simulink model "Example3_Calibrating_The_AR_Drone"  (R2016a)
settings: configuration reference "AR_Drone_ConfigSet" (kept outside this file)
undefined symbols (not defined in the file or in its folder): Accel_Calib_Gain, Accel_Calib_Offset, DiscIntNeverNeededParam, Mag_Calib_Gain_Vector, Mag_Calib_Offset_Vector
libraries: simulink x5, vrlib x2, AR_Drone_2_Library x1
(part 1 of 2)
settings Model: SimulationMode=external  Creator=sannem  LastModifiedBy=sannem
settings ConfigSetRef: SourceLocation=Base Workspace

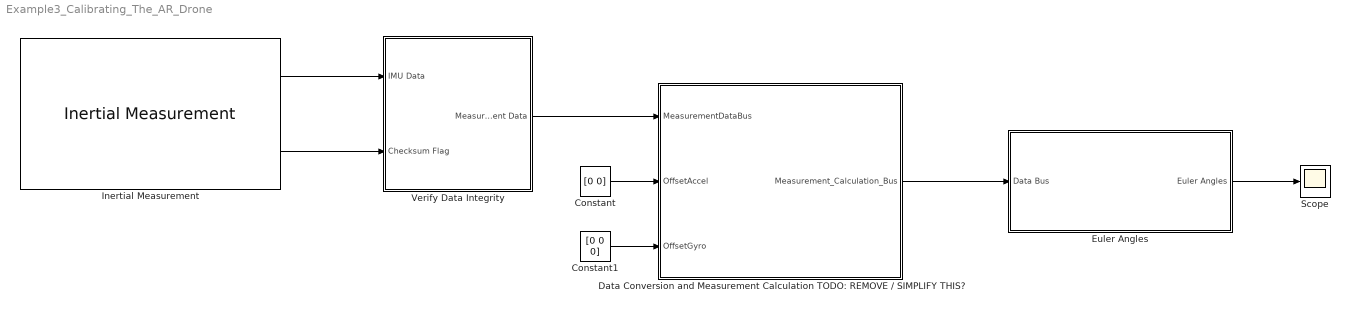
== system Example3_Calibrating_The_AR_Drone ==
  Constant : Constant  Value=[0 0]
  Constant1 : Constant  Value=[0 0 0]
  Data Conversion and Measurement Calculation TODO: REMOVE / SIMPLIFY THIS? : Subsystem
  Euler Angles : Subsystem
  Inertial Measurement : AR_Drone_2_Library/Inertial Measurement  Ts=1/400
  Scope : Scope
  Verify Data Integrity : Subsystem
  wires:
  Euler Angles/1(Euler Angles) -> Scope/1
  Constant/1 -> Data Conversion and Measurement Calculation TODO: REMOVE / SIMPLIFY THIS?/2(OffsetAccel)
  Data Conversion and Measurement Calculation TODO: REMOVE / SIMPLIFY THIS?/1(Measurement_Calculation_Bus) -> Euler Angles/1(Data Bus)
  Constant1/1 -> Data Conversion and Measurement Calculation TODO: REMOVE / SIMPLIFY THIS?/3(OffsetGyro)
  Inertial Measurement/1 -> Verify Data Integrity/1(IMU Data)
  Inertial Measurement/2 -> Verify Data Integrity/2(Checksum Flag)
  Verify Data Integrity/1(Measurement Data) -> Data Conversion and Measurement Calculation TODO: REMOVE / SIMPLIFY THIS?/1(MeasurementDataBus)

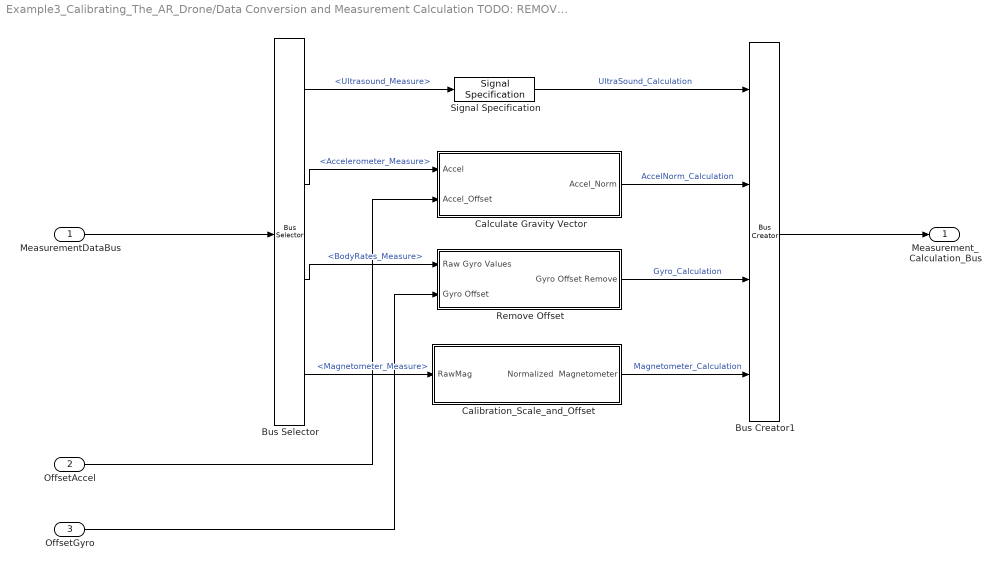
== system Example3_Calibrating_The_AR_Drone/Data Conversion and Measurement Calculation TODO: REMOVE // SIMPLIFY THIS? ==
  MeasurementDataBus : Inport
  OffsetAccel : Inport  Port=2
  OffsetGyro : Inport  Port=3
  Bus Creator1 : BusCreator  Inputs=4
  Bus Selector : BusSelector  OutputSignals=Ultrasound_Measure,Accelerometer_Measure,BodyRates_Measure,Magnetometer_Measure
  Calculate Gravity Vector : Subsystem
  Calibration_Scale_and_Offset : Subsystem
  Remove Offset : Subsystem
  Signal Specification : SignalSpecification
  Measurement_Calculation_Bus : Outport
  wires:
  MeasurementDataBus/1 -> Bus Selector/1
  Bus Selector/4 -> Calibration_Scale_and_Offset/1(RawMag)  "<Magnetometer_Measure>"
  OffsetAccel/1 -> Calculate Gravity Vector/2(Accel_Offset)
  OffsetGyro/1 -> Remove Offset/2(Gyro Offset)
  Bus Selector/3 -> Remove Offset/1(Raw Gyro Values)  "<BodyRates_Measure>"
  Bus Selector/1 -> Signal Specification/1  "<Ultrasound_Measure>"
  Calibration_Scale_and_Offset/1(Normalized  Magnetometer) -> Bus Creator1/4  "Magnetometer_Calculation"
  Remove Offset/1(Gyro Offset Remove) -> Bus Creator1/3  "Gyro_Calculation"
  Signal Specification/1 -> Bus Creator1/1  "UltraSound_Calculation"
  Calculate Gravity Vector/1(Accel_Norm) -> Bus Creator1/2  "AccelNorm_Calculation"
  Bus Creator1/1 -> Measurement_Calculation_Bus/1
  Bus Selector/2 -> Calculate Gravity Vector/1(Accel)  "<Accelerometer_Measure>"

== system Example3_Calibrating_The_AR_Drone/Euler Angles ==
  Data Bus : Inport  OutDataTypeStr=Bus: Measurement_Calculation_Bus
  Bus Selector2 : BusSelector  OutputSignals=AccelNorm_Calculation
  Bus Selector3 : BusSelector  OutputSignals=Gyro_Calculation
  Compute Euler Angles : Subsystem
  Invert : Gain  Gain=-1
  Mux : Mux  Inputs=3
  Euler Angles : Outport
  wires:
  Data Bus/1 -> Bus Selector3/1, Bus Selector2/1
  Bus Selector3/1 -> Compute Euler Angles/2(Gyroscope Data)  "<Gyro_Calculation>"
  Bus Selector2/1 -> Compute Euler Angles/1(Accelerometer Data)  "<AccelNorm_Calculation>"
  Compute Euler Angles/1(Filtered Roll) -> Mux/1
  Compute Euler Angles/2(Filtered Pitch) -> Mux/2
  Compute Euler Angles/3(Yaw) -> Mux/3
  Mux/1 -> Invert/1
  Invert/1 -> Euler Angles/1

== system Example3_Calibrating_The_AR_Drone/Verify Data Integrity ==
  IMU Data : Inport
  Checksum Flag : Inport  Port=2
  Bus Creator1 : BusCreator  Inputs=5
  CheckSum Pre-Processing : Subsystem  TreatAsAtomicUnit=on
      settings: RTWSystemCode=Inline
  Measurement Data : Outport
  wires:
  CheckSum Pre-Processing/2(Magnetometer_Measure) -> Bus Creator1/2  "Magnetometer_Measure"
  Bus Creator1/1 -> Measurement Data/1  "RawMeasurement_DataBus"
  CheckSum Pre-Processing/3(BodyRates_Measure) -> Bus Creator1/3  "BodyRates_Measure"
  CheckSum Pre-Processing/1(UltraSoundHeight_Measure) -> Bus Creator1/1  "Ultrasound_Measure"
  Checksum Flag/1 -> CheckSum Pre-Processing/2(CheckSumFlag)
  IMU Data/1 -> CheckSum Pre-Processing/1(IMU Packets)
  CheckSum Pre-Processing/5(GyroTemp_Measure) -> Bus Creator1/5  "GyroTemp_Measure"
  CheckSum Pre-Processing/4(Accelerometer_Measure) -> Bus Creator1/4  "Accelerometer_Measure"

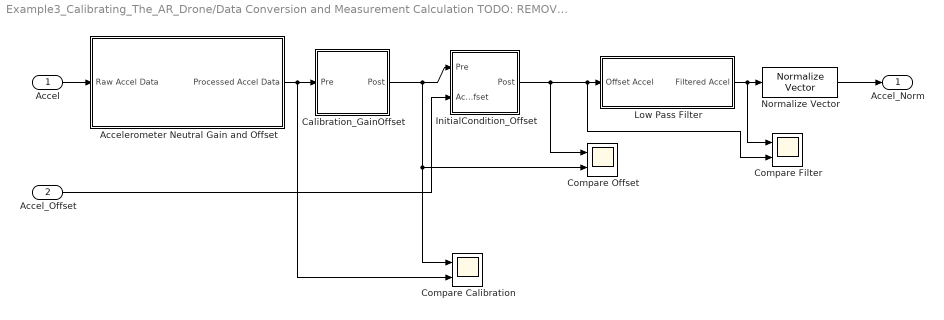
== system Example3_Calibrating_The_AR_Drone/Data Conversion and Measurement Calculation TODO: REMOVE // SIMPLIFY THIS?/Calculate Gravity Vector ==
  Accel : Inport
  Accel_Offset : Inport  Port=2
  Accelerometer Neutral Gain and Offset : Subsystem
  Calibration_GainOffset : Subsystem
  Compare Calibration : Scope  NumInputPorts=2
  Compare Filter : Scope  NumInputPorts=2
  Compare Offset : Scope  NumInputPorts=2
  InitialCondition_Offset : Subsystem
  Low Pass Filter : Subsystem
  Normalize Vector : vrlib/Utilities/Normalize Vector  maxzero=0
  Accel_Norm : Outport
  wires:
  Accel_Offset/1 -> InitialCondition_Offset/2(Accel_Offset)
  Accelerometer Neutral Gain and Offset/1(Processed Accel Data) -> Compare Calibration/2, Calibration_GainOffset/1(Pre)
  Calibration_GainOffset/1(Post) -> Compare Offset/2, Compare Calibration/1, InitialCondition_Offset/1(Pre)
  Low Pass Filter/1(Filtered Accel) -> Normalize Vector/1, Compare Filter/1
  InitialCondition_Offset/1(Post) -> Low Pass Filter/1(Offset Accel), Compare Filter/2, Compare Offset/1
  Accel/1 -> Accelerometer Neutral Gain and Offset/1(Raw Accel Data)
  Normalize Vector/1 -> Accel_Norm/1

== system Example3_Calibrating_The_AR_Drone/Data Conversion and Measurement Calculation TODO: REMOVE // SIMPLIFY THIS?/Calibration_Scale_and_Offset ==
  RawMag : Inport
  Normalize Vector : vrlib/Utilities/Normalize Vector  maxzero=0
  Process Raw Mag Data : Subsystem  Variant=on  OverrideUsingVariant=TempVariantA
  Normalized  Magnetometer : Outport
  wires:
  Process Raw Mag Data/1(MagVector) -> Normalize Vector/1
  RawMag/1 -> Process Raw Mag Data/1(Magnetometer)
  Normalize Vector/1 -> Normalized  Magnetometer/1

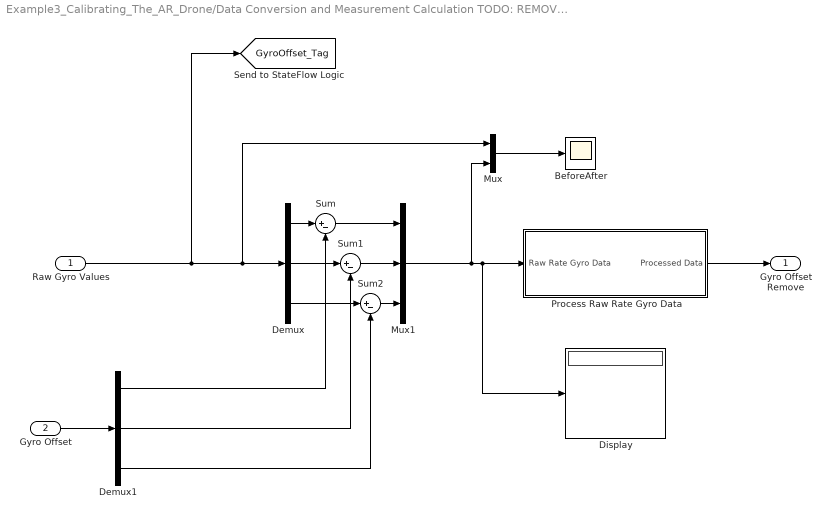
== system Example3_Calibrating_The_AR_Drone/Data Conversion and Measurement Calculation TODO: REMOVE // SIMPLIFY THIS?/Remove Offset ==
  Raw Gyro Values : Inport
  Gyro Offset : Inport  Port=2
  BeforeAfter : Scope
  Demux : Demux  Outputs=3
  Demux1 : Demux  Outputs=3
  Display : Display
  Mux : Mux  Inputs=2
  Mux1 : Mux  Inputs=3
  Process Raw Rate Gyro Data : Subsystem
  Sum : Sum  Inputs=|+-
  Sum1 : Sum  Inputs=|+-
  Sum2 : Sum  Inputs=|+-
  Gyro Offset Remove : Outport
  tag scope: GyroOffset_Tag=global
  wires:
  Process Raw Rate Gyro Data/1(Processed Data) -> Gyro Offset Remove/1
  Mux/1 -> BeforeAfter/1
  Raw Gyro Values/1 -> Demux/1, Mux/1, [GyroOffset_Tag]
  Gyro Offset/1 -> Demux1/1
  Mux1/1 -> Process Raw Rate Gyro Data/1(Raw Rate Gyro Data), Display/1, Mux/2
  Demux1/3 -> Sum2/2
  Demux1/2 -> Sum1/2
  Demux1/1 -> Sum/2
  Demux/2 -> Sum1/1
  Demux/1 -> Sum/1
  Sum1/1 -> Mux1/2
  Demux/3 -> Sum2/1
  Sum2/1 -> Mux1/3
  Sum/1 -> Mux1/1

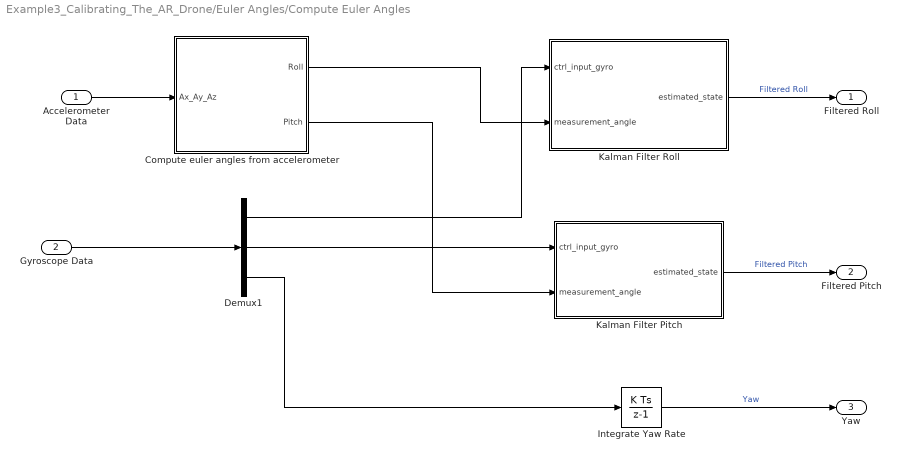
== system Example3_Calibrating_The_AR_Drone/Euler Angles/Compute Euler Angles ==
  Accelerometer Data : Inport
  Gyroscope Data : Inport  Port=2
  Compute euler angles from accelerometer : MATLAB Function  TreatAsAtomicUnit=on
  Demux1 : Demux  Outputs=3
  Integrate Yaw Rate : DiscreteIntegrator  SampleTime=1/400  OutDataTypeStr=double  ICPrevOutput=DiscIntNeverNeededParam  ICPrevScaledInput=DiscIntNeverNeededParam
  Kalman Filter Pitch : MATLAB Function  TreatAsAtomicUnit=on
  Kalman Filter Roll : MATLAB Function  TreatAsAtomicUnit=on
  Filtered Roll : Outport
  Filtered Pitch : Outport  Port=2
  Yaw : Outport  Port=3
  wires:
  Compute euler angles from accelerometer/2(Pitch) -> Kalman Filter Pitch/2(measurement_angle)
  Integrate Yaw Rate/1 -> Yaw/1  "Yaw"
  Kalman Filter Roll/1(estimated_state) -> Filtered Roll/1  "Filtered Roll"
  Demux1/3 -> Integrate Yaw Rate/1
  Demux1/2 -> Kalman Filter Pitch/1(ctrl_input_gyro)
  Kalman Filter Pitch/1(estimated_state) -> Filtered Pitch/1  "Filtered Pitch"
  Demux1/1 -> Kalman Filter Roll/1(ctrl_input_gyro)
  Compute euler angles from accelerometer/1(Roll) -> Kalman Filter Roll/2(measurement_angle)
  Accelerometer Data/1 -> Compute euler angles from accelerometer/1(Ax_Ay_Az)
  Gyroscope Data/1 -> Demux1/1

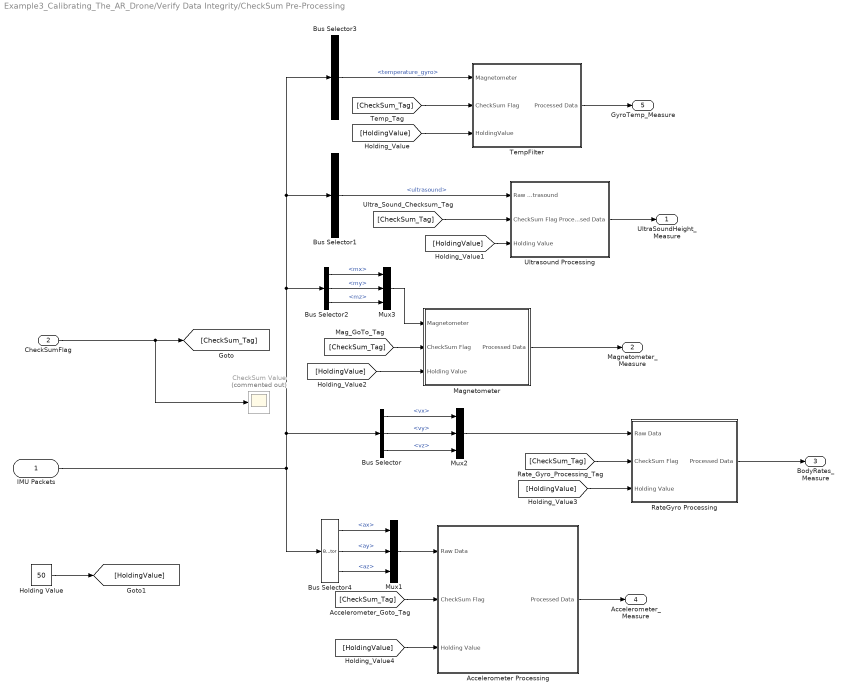
== system Example3_Calibrating_The_AR_Drone/Verify Data Integrity/CheckSum Pre-Processing ==
  IMU Packets : Inport
  CheckSumFlag : Inport  Port=2
  Accelerometer Processing : Subsystem
  Bus Selector : BusSelector  OutputSignals=vx,vy,vz
  Bus Selector1 : BusSelector  OutputSignals=ultrasound
  Bus Selector2 : BusSelector  OutputSignals=mx,my,mz
  Bus Selector3 : BusSelector  OutputSignals=temperature_gyro
  Bus Selector4 : BusSelector  OutputSignals=ax,ay,az
  CheckSum Value : Scope  Commented=on
  Holding Value : Constant  Value=50
  Magnetometer : Subsystem
  Mux1 : Mux  Inputs=3
  Mux2 : Mux  Inputs=3
  Mux3 : Mux  Inputs=3
  RateGyro Processing : Subsystem
  TempFilter : Subsystem
  Ultrasound Processing : Subsystem
  UltraSoundHeight_Measure : Outport
  Magnetometer_Measure : Outport  Port=2
  BodyRates_Measure : Outport  Port=3
  Accelerometer_Measure : Outport  Port=4
  GyroTemp_Measure : Outport  Port=5
  wires:
  Mux3/1 -> Magnetometer/1(Magnetometer)
  Holding Value/1 -> [HoldingValue]
  [HoldingValue] -> Accelerometer Processing/3(Holding Value)
  [HoldingValue] -> RateGyro Processing/3(Holding Value)
  [HoldingValue] -> Magnetometer/3(Holding Value)
  [HoldingValue] -> Ultrasound Processing/3(Holding Value)
  [HoldingValue] -> TempFilter/3(HoldingValue)
  [CheckSum_Tag] -> TempFilter/2(CheckSum Flag)
  TempFilter/1(Processed Data) -> GyroTemp_Measure/1
  Bus Selector3/1 -> TempFilter/1(Magnetometer)  "<temperature_gyro>"
  Bus Selector/3 -> Mux2/3  "<vz>"
  Bus Selector/2 -> Mux2/2  "<vy>"
  Bus Selector/1 -> Mux2/1  "<vx>"
  Ultrasound Processing/1(Processed Data) -> UltraSoundHeight_Measure/1
  [CheckSum_Tag] -> Accelerometer Processing/2(CheckSum Flag)
  Magnetometer/1(Processed Data) -> Magnetometer_Measure/1
  [CheckSum_Tag] -> Magnetometer/2(CheckSum Flag)
  Bus Selector2/3 -> Mux3/3  "<mz>"
  Bus Selector2/2 -> Mux3/2  "<my>"
  Bus Selector2/1 -> Mux3/1  "<mx>"
  RateGyro Processing/1(Processed Data) -> BodyRates_Measure/1
  [CheckSum_Tag] -> RateGyro Processing/2(CheckSum Flag)
  Mux2/1 -> RateGyro Processing/1(Raw Data)
  Accelerometer Processing/1(Processed Data) -> Accelerometer_Measure/1
  [CheckSum_Tag] -> Ultrasound Processing/2(CheckSum Flag)
  Mux1/1 -> Accelerometer Processing/1(Raw Data)
  Bus Selector4/3 -> Mux1/3  "<az>"
  Bus Selector4/2 -> Mux1/2  "<ay>"
  Bus Selector4/1 -> Mux1/1  "<ax>"
  IMU Packets/1 -> Bus Selector4/1, Bus Selector2/1, Bus Selector1/1, Bus Selector3/1, Bus Selector/1
  CheckSumFlag/1 -> CheckSum Value/1, [CheckSum_Tag]
  Bus Selector1/1 -> Ultrasound Processing/1(Raw Ultrasound)  "<ultrasound>"

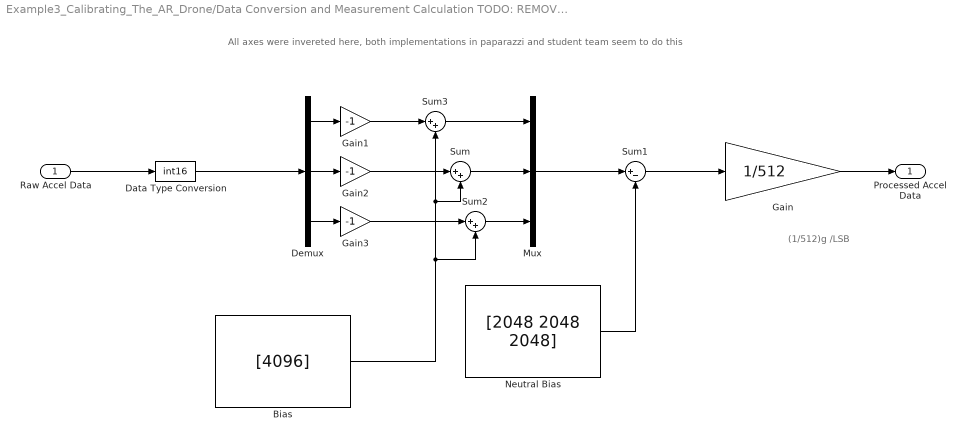
== system Example3_Calibrating_The_AR_Drone/Data Conversion and Measurement Calculation TODO: REMOVE // SIMPLIFY THIS?/Calculate Gravity Vector/Accelerometer Neutral Gain and Offset ==
  note: (1/512)g /LSB
  note: All axes were invereted here, both implementations in paparazzi and student team seem to do this
  Raw Accel Data : Inport
  Bias : Constant  Value=[4096]
  Data Type Conversion : DataTypeConversion  OutDataTypeStr=int16
  Demux : Demux  Outputs=3
  Gain : Gain  Gain=1/512
  Gain1 : Gain  Gain=-1  OutDataTypeStr=double
  Gain2 : Gain  Gain=-1  OutDataTypeStr=double
  Gain3 : Gain  Gain=-1  OutDataTypeStr=double
  Mux : Mux  Inputs=3
  Neutral Bias : Constant  Value=[2048 2048 2048]
  Sum : Sum  Inputs=|++
  Sum1 : Sum  Inputs=|+-
  Sum2 : Sum  Inputs=|++
  Sum3 : Sum  Inputs=|++
  Processed Accel Data : Outport
  wires:
  Gain1/1 -> Sum3/1
  Data Type Conversion/1 -> Demux/1
  Bias/1 -> Sum3/2, Sum/2, Sum2/2
  Sum2/1 -> Mux/3
  Gain3/1 -> Sum2/1
  Demux/3 -> Gain3/1
  Sum/1 -> Mux/2
  Gain2/1 -> Sum/1
  Demux/2 -> Gain2/1
  Sum3/1 -> Mux/1
  Demux/1 -> Gain1/1
  Raw Accel Data/1 -> Data Type Conversion/1
  Neutral Bias/1 -> Sum1/2
  Mux/1 -> Sum1/1
  Gain/1 -> Processed Accel Data/1
  Sum1/1 -> Gain/1

== system Example3_Calibrating_The_AR_Drone/Data Conversion and Measurement Calculation TODO: REMOVE // SIMPLIFY THIS?/Calculate Gravity Vector/Calibration_GainOffset ==
  Pre : Inport
  Accel_Calib_Gain : Constant  Value=[Accel_Calib_Gain.Gain_X Accel_Calib_Gain.Gain_Y Accel_Calib_Gain.Gain_Z]
      settings: AttributesFormatString=%<Value>
  Accel_Calib_Offset : Constant  Value="[Accel_Calib_Offset.Gain_X  Accel_Calib_Offset.Gain_Y  Accel_Calib_Offset.Gain_Z]"
      settings: AttributesFormatString=%<Value>
  Gain : Gain  Gain=-1  OutDataTypeStr=Inherit: Same as input
  Multiply : Product  Inputs=*/
  Sum : Sum  Inputs=|+-
  Post : Outport
  wires:
  Gain/1 -> Multiply/2
  Accel_Calib_Gain/1 -> Gain/1
  Pre/1 -> Sum/1
  Sum/1 -> Multiply/1
  Accel_Calib_Offset/1 -> Sum/2
  Multiply/1 -> Post/1

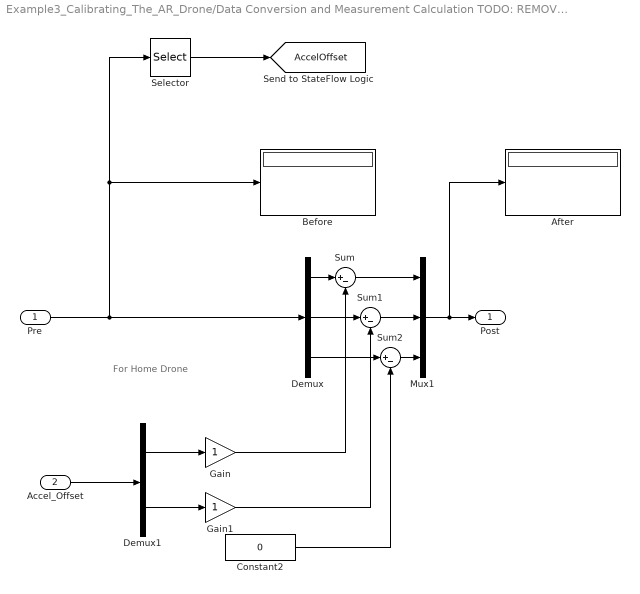
== system Example3_Calibrating_The_AR_Drone/Data Conversion and Measurement Calculation TODO: REMOVE // SIMPLIFY THIS?/Calculate Gravity Vector/InitialCondition_Offset ==
  note: For Home Drone
  Pre : Inport
  Accel_Offset : Inport  Port=2
  After : Display
  Before : Display
  Constant2 : Constant  Value=0
  Demux : Demux  Outputs=3
  Demux1 : Demux  Outputs=2
  Gain : Gain
  Gain1 : Gain
  Mux1 : Mux  Inputs=3
  Selector : Selector  InputPortWidth=3  IndexOptions=Index vector (dialog)  Indices=[1 2]  OutputSizes=1
  Sum : Sum  Inputs=|+-
  Sum1 : Sum  Inputs=|+-
  Sum2 : Sum  Inputs=|+-
  Post : Outport
  tag scope: AccelOffset=global
  wires:
  Constant2/1 -> Sum2/2
  Gain1/1 -> Sum1/2
  Gain/1 -> Sum/2
  Selector/1 -> [AccelOffset]
  Pre/1 -> Before/1, Selector/1, Demux/1
  Demux1/2 -> Gain1/1
  Demux1/1 -> Gain/1
  Accel_Offset/1 -> Demux1/1
  Mux1/1 -> After/1, Post/1
  Demux/2 -> Sum1/1
  Demux/1 -> Sum/1
  Sum1/1 -> Mux1/2
  Demux/3 -> Sum2/1
  Sum2/1 -> Mux1/3
  Sum/1 -> Mux1/1

== system Example3_Calibrating_The_AR_Drone/Data Conversion and Measurement Calculation TODO: REMOVE // SIMPLIFY THIS?/Calculate Gravity Vector/Low Pass Filter ==
  Offset Accel : Inport
  Add : Sum
  Gain : Gain  Gain=0.8
  Gain1 : Gain  Gain=0.2
  Unit Delay : UnitDelay  SampleTime=-1
  Filtered Accel : Outport
  wires:
  Offset Accel/1 -> Gain1/1
  Add/1 -> Filtered Accel/1, Unit Delay/1
  Gain/1 -> Add/2
  Gain1/1 -> Add/1
  Unit Delay/1 -> Gain/1

== system Example3_Calibrating_The_AR_Drone/Data Conversion and Measurement Calculation TODO: REMOVE // SIMPLIFY THIS?/Calibration_Scale_and_Offset/Process Raw Mag Data ==
  Magnetometer : Inport
  Process Raw Mag Data (Home_330453) : Subsystem  VariantControl=TempVariantA
  Process Raw Mag Data (Work_255725) : Subsystem  VariantControl=TempVariantB
  MagVector : Outport

== system Example3_Calibrating_The_AR_Drone/Data Conversion and Measurement Calculation TODO: REMOVE // SIMPLIFY THIS?/Remove Offset/Process Raw Rate Gyro Data ==
  note: const float Sensitivity[ 3 ] = { 0.0609 , 0.0609 , 0.0609 } ;
      | const float Neutral[ 3 ] = { 0.0 , 0.0 , 0.0 } ;
      | const int16_t Offset[ 3 ] = { - 73 , 14 , - 13 } ;
      | const int16_t Noises[ 3 ] = { 35 , 35 , 15 } ;
      |
      | int16_t vRaws[ 3 ] = {
      | Navdata :: IMU :: Gyroscope :: getRawX (),
      | Navdata :: IMU :: Gyroscope :: getRawY (),
      | Navdata :: IMU :: Gyroscope :: getRawZ ()
      | } ;
      |
      | gyroscope[i] = vRaws[i] * Gyroscope :: Sensitivity[i] * M_PI / 180.0 ;
  Raw Rate Gyro Data : Inport
  Gain : Gain  Gain=[0.0609, 0.0609, 0.0609]  ParamDataTypeStr=double
  Processed Data : Outport
  wires:
  Gain/1 -> Processed Data/1
  Raw Rate Gyro Data/1 -> Gain/1

== system Example3_Calibrating_The_AR_Drone/Verify Data Integrity/CheckSum Pre-Processing/Accelerometer Processing ==
  Raw Data : Inport
  CheckSum Flag : Inport  Port=2
  Holding Value : Inport  Port=3
  Calculate Accel Data : Subsystem  Commented=through
  CheckSum Correction : Subsystem
  Processed Data : Outport
  wires:
  Holding Value/1 -> CheckSum Correction/3(Holding Value)
  Calculate Accel Data/1(Processed Accel Data) -> CheckSum Correction/1(CalculatedData)
  CheckSum Correction/1(Pre-Processed Height) -> Processed Data/1
  Raw Data/1 -> Calculate Accel Data/1(Raw Accel Data)
  CheckSum Flag/1 -> CheckSum Correction/2(CheckSumFlag)

== system Example3_Calibrating_The_AR_Drone/Verify Data Integrity/CheckSum Pre-Processing/Magnetometer ==
  Magnetometer : Inport
  CheckSum Flag : Inport  Port=2
  Holding Value : Inport  Port=3
  CheckSum Correction : Subsystem
  Process Raw Mag Data : Subsystem  Commented=through
  Processed Data : Outport
  wires:
  Holding Value/1 -> CheckSum Correction/3(Holding Value)
  Process Raw Mag Data/1(ProcessedData) -> CheckSum Correction/1(CalculatedData)
  Magnetometer/1 -> Process Raw Mag Data/1(Magnetometer)
  CheckSum Correction/1(Pre-Processed Data) -> Processed Data/1
  CheckSum Flag/1 -> CheckSum Correction/2(CheckSumFlag)

== system Example3_Calibrating_The_AR_Drone/Verify Data Integrity/CheckSum Pre-Processing/RateGyro Processing ==
  Raw Data : Inport
  CheckSum Flag : Inport  Port=2
  Holding Value : Inport  Port=3
  CheckSum Correction : Subsystem
  Process Data : Subsystem  Commented=through
  Processed Data : Outport
  wires:
  Holding Value/1 -> CheckSum Correction/3(Holding Value)
  Process Data/1(Processed Data) -> CheckSum Correction/1(CalculatedData)
  Raw Data/1 -> Process Data/1(Raw Data)
  CheckSum Correction/1(Pre-Processed Height) -> Processed Data/1
  CheckSum Flag/1 -> CheckSum Correction/2(CheckSumFlag)

== system Example3_Calibrating_The_AR_Drone/Verify Data Integrity/CheckSum Pre-Processing/TempFilter ==
  Magnetometer : Inport
  CheckSum Flag : Inport  Port=2
  HoldingValue : Inport  Port=3
  CheckSum Correction : Subsystem
  Process Raw Mag Data : Subsystem  Commented=through
  Processed Data : Outport
  wires:
  HoldingValue/1 -> CheckSum Correction/3(Holding Value)
  Process Raw Mag Data/1(ProcessedData) -> CheckSum Correction/1(CalculatedData)
  Magnetometer/1 -> Process Raw Mag Data/1(Magnetometer)
  CheckSum Correction/1(Pre-Processed Data) -> Processed Data/1
  CheckSum Flag/1 -> CheckSum Correction/2(CheckSumFlag)

== system Example3_Calibrating_The_AR_Drone/Verify Data Integrity/CheckSum Pre-Processing/Ultrasound Processing ==
  note: '192.168.1.1' 1 17725
  Raw Ultrasound : Inport
  CheckSum Flag : Inport  Port=2
  Holding Value : Inport  Port=3
  CheckSum Correction : Subsystem
  Data Type Conversion1 : DataTypeConversion
  Delay1 : Delay  DelayLength=1  InitialCondition=0
  Height Calculation : MATLAB Function  TreatAsAtomicUnit=on
  Saturation1 : Saturate  UpperLimit=100e3  LowerLimit=0
  Processed Data : Outport
  wires:
  Holding Value/1 -> CheckSum Correction/3(Holding Value)
  Saturation1/1 -> Processed Data/1
  CheckSum Correction/1(Pre-Processed Height) -> Saturation1/1
  CheckSum Flag/1 -> CheckSum Correction/2(CheckSumFlag)
  Height Calculation/1(y) -> CheckSum Correction/1(CalculatedData)
  Raw Ultrasound/1 -> Data Type Conversion1/1
  Height Calculation/2(prev_good_height) -> Delay1/1
  Data Type Conversion1/1 -> Height Calculation/1(u)
  Delay1/1 -> Height Calculation/2(z_1)

== system Example3_Calibrating_The_AR_Drone/Data Conversion and Measurement Calculation TODO: REMOVE // SIMPLIFY THIS?/Calibration_Scale_and_Offset/Process Raw Mag Data/Process Raw Mag Data (Home_330453) ==
  note: magnetometer[ 0 ] = - ( float ) navdata.mx ;
      | magnetometer[ 1 ] = ( float ) navdata.my ;
      | magnetometer[ 2 ] = - ( float ) navdata.mz ;
      | const float Sensitivity[ 3 ] = { 0.0071492608 , 0.0070882491 , 0.0074057781 } ;
      | const float Neutral[ 3 ] = { 118.0 , - 65.0 , 110.0 } ;
  Magnetometer : Inport
  Bias : Constant  Commented=on  Value=[-23 4.3 1.44]
  Constant : Constant  Value=[Mag_Calib_Offset_Vector.Gain_X Mag_Calib_Offset_Vector.Gain_Y Mag_Calib_Offset_Vector.Gain_Z]
      settings: AttributesFormatString=%<Value>
  Constant1 : Constant  Value=[Mag_Calib_Gain_Vector.Gain_X Mag_Calib_Gain_Vector.Gain_Y Mag_Calib_Gain_Vector.Gain_Z]
      settings: AttributesFormatString=%<Value>
  Divide : Product  Inputs=/*
  Sum : Sum  Inputs=|+-
  postGain : Gain  Commented=on  Gain=1./[187 163 139]
  MagVector : Outport
  wires:
  Constant1/1 -> Divide/1
  Sum/1 -> Divide/2
  Magnetometer/1 -> Sum/1
  Constant/1 -> Sum/2
  Divide/1 -> MagVector/1

== system Example3_Calibrating_The_AR_Drone/Data Conversion and Measurement Calculation TODO: REMOVE // SIMPLIFY THIS?/Calibration_Scale_and_Offset/Process Raw Mag Data/Process Raw Mag Data (Work_255725) ==
  note: 158 145 136
  note: magnetometer[ 0 ] = - ( float ) navdata.mx ;
      | magnetometer[ 1 ] = ( float ) navdata.my ;
      | magnetometer[ 2 ] = - ( float ) navdata.mz ;
      | const float Sensitivity[ 3 ] = { 0.0071492608 , 0.0070882491 , 0.0074057781 } ;
      | const float Neutral[ 3 ] = { 118.0 , - 65.0 , 110.0 } ;
  Magnetometer : Inport
  Bias : Constant  Value=[2.93 18.9 77.5]
  Low Pass Filter1 : Subsystem  Commented=through
      mask Display: disp(['Elliptic Filter with 20 Hz corner', '\n', '44 dB stopband.'])
  Sum : Sum  Inputs=|+-
  postGain : Gain  Gain=1./[167 135 132]
  preGain : Gain  Commented=through  Gain=[1 1 1]
  MagVector : Outport
  wires:
  postGain/1 -> Low Pass Filter1/1(Input)
  Magnetometer/1 -> preGain/1
  Sum/1 -> postGain/1
  preGain/1 -> Sum/1
  Bias/1 -> Sum/2
  Low Pass Filter1/1(Output) -> MagVector/1

== system Example3_Calibrating_The_AR_Drone/Verify Data Integrity/CheckSum Pre-Processing/Accelerometer Processing/Calculate Accel Data ==
  Raw Accel Data : Inport
  Bias : Constant  Value=[0 4096 4096]
  Gain : Gain  Gain=[0.001953125, 0.001953125, 0.001953125]
  Neutral Bias : Constant  Value=[2048 2048 2048]
  Sum : Sum  Inputs=|-+
  Sum1 : Sum  Inputs=|+-
  Processed Accel Data : Outport
  wires:
  Bias/1 -> Sum/2
  Neutral Bias/1 -> Sum1/2
  Sum/1 -> Sum1/1
  Gain/1 -> Processed Accel Data/1
  Sum1/1 -> Gain/1
  Raw Accel Data/1 -> Sum/1

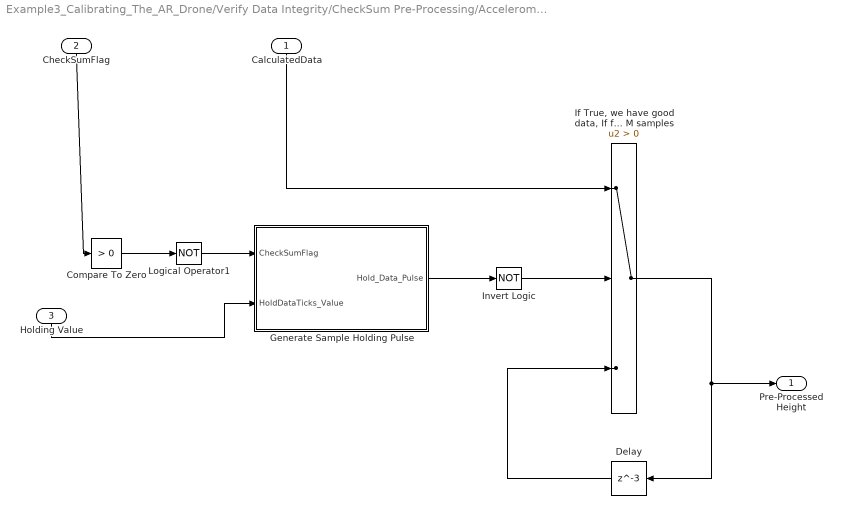
== system Example3_Calibrating_The_AR_Drone/Verify Data Integrity/CheckSum Pre-Processing/Accelerometer Processing/CheckSum Correction ==
  CalculatedData : Inport
  CheckSumFlag : Inport  Port=2
  Holding Value : Inport  Port=3
  Compare To Zero : simulink/Logic and Bit Operations/Compare To Zero  relop=>  OutDataTypeStr=boolean
  Delay : Delay  DelayLength=3  InitialCondition=0
  Generate Sample Holding Pulse : Subsystem
  "If True, we have good data, If false, we have bad data, With bad data, use previous good data from N samples ago and hold it on that value for M samples" : Switch  Criteria=u2 > Threshold
  Invert Logic : Logic  Operator=NOT  AllPortsSameDT=off  OutDataTypeStr=boolean
  Logical Operator1 : Logic  Operator=NOT  AllPortsSameDT=off  OutDataTypeStr=boolean
  Pre-Processed Height : Outport
  wires:
  Holding Value/1 -> Generate Sample Holding Pulse/2(HoldDataTicks_Value)
  Invert Logic/1 -> "If True, we have good data, If false, we have bad data, With bad data, use previous good data from N samples ago and hold it on that value for M samples"/2
  Logical Operator1/1 -> Generate Sample Holding Pulse/1(CheckSumFlag)
  Generate Sample Holding Pulse/1(Hold_Data_Pulse) -> Invert Logic/1
  Compare To Zero/1 -> Logical Operator1/1
  Delay/1 -> "If True, we have good data, If false, we have bad data, With bad data, use previous good data from N samples ago and hold it on that value for M samples"/3
  "If True, we have good data, If false, we have bad data, With bad data, use previous good data from N samples ago and hold it on that value for M samples"/1 -> Delay/1, Pre-Processed Height/1
  CalculatedData/1 -> "If True, we have good data, If false, we have bad data, With bad data, use previous good data from N samples ago and hold it on that value for M samples"/1
  CheckSumFlag/1 -> Compare To Zero/1

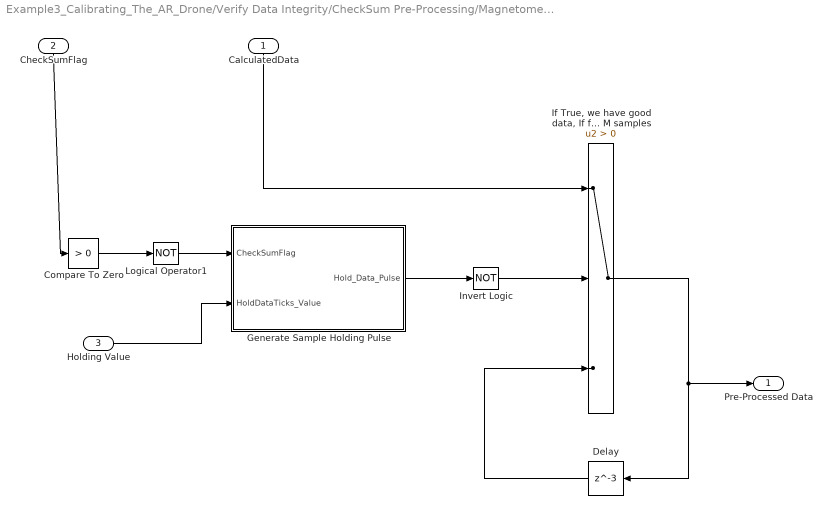
== system Example3_Calibrating_The_AR_Drone/Verify Data Integrity/CheckSum Pre-Processing/Magnetometer/CheckSum Correction ==
  CalculatedData : Inport
  CheckSumFlag : Inport  Port=2
  Holding Value : Inport  Port=3
  Compare To Zero : simulink/Logic and Bit Operations/Compare To Zero  relop=>  OutDataTypeStr=boolean
  Delay : Delay  DelayLength=3  InitialCondition=0
  Generate Sample Holding Pulse : Subsystem
  "If True, we have good data, If false, we have bad data, With bad data, use previous good data from N samples ago and hold it on that value for M samples" : Switch  Criteria=u2 > Threshold
  Invert Logic : Logic  Operator=NOT  AllPortsSameDT=off  OutDataTypeStr=boolean
  Logical Operator1 : Logic  Operator=NOT  AllPortsSameDT=off  OutDataTypeStr=boolean
  Pre-Processed Data : Outport
  wires:
  Holding Value/1 -> Generate Sample Holding Pulse/2(HoldDataTicks_Value)
  Invert Logic/1 -> "If True, we have good data, If false, we have bad data, With bad data, use previous good data from N samples ago and hold it on that value for M samples"/2
  Logical Operator1/1 -> Generate Sample Holding Pulse/1(CheckSumFlag)
  Generate Sample Holding Pulse/1(Hold_Data_Pulse) -> Invert Logic/1
  Compare To Zero/1 -> Logical Operator1/1
  Delay/1 -> "If True, we have good data, If false, we have bad data, With bad data, use previous good data from N samples ago and hold it on that value for M samples"/3
  "If True, we have good data, If false, we have bad data, With bad data, use previous good data from N samples ago and hold it on that value for M samples"/1 -> Delay/1, Pre-Processed Data/1
  CalculatedData/1 -> "If True, we have good data, If false, we have bad data, With bad data, use previous good data from N samples ago and hold it on that value for M samples"/1
  CheckSumFlag/1 -> Compare To Zero/1

== system Example3_Calibrating_The_AR_Drone/Verify Data Integrity/CheckSum Pre-Processing/Magnetometer/Process Raw Mag Data ==
  note: magnetometer[ 0 ] = - ( float ) navdata.mx ;
      | magnetometer[ 1 ] = ( float ) navdata.my ;
      | magnetometer[ 2 ] = - ( float ) navdata.mz ;
      | const float Sensitivity[ 3 ] = { 0.0071492608 , 0.0070882491 , 0.0074057781 } ;
      | const float Neutral[ 3 ] = { 118.0 , - 65.0 , 110.0 } ;
  Magnetometer : Inport
  Bias : Constant  Value=[ 118.0, -65.0, 110.0 ]
  Sum : Sum  Inputs=|+-
  postGain : Gain  Gain=[0.0071492608, 0.0070882491, 0.0074057781]
  preGain : Gain  Gain=[-1 1 -1]
  ProcessedData : Outport
  wires:
  Bias/1 -> Sum/2
  preGain/1 -> Sum/1
  Sum/1 -> postGain/1
  Magnetometer/1 -> preGain/1
  postGain/1 -> ProcessedData/1

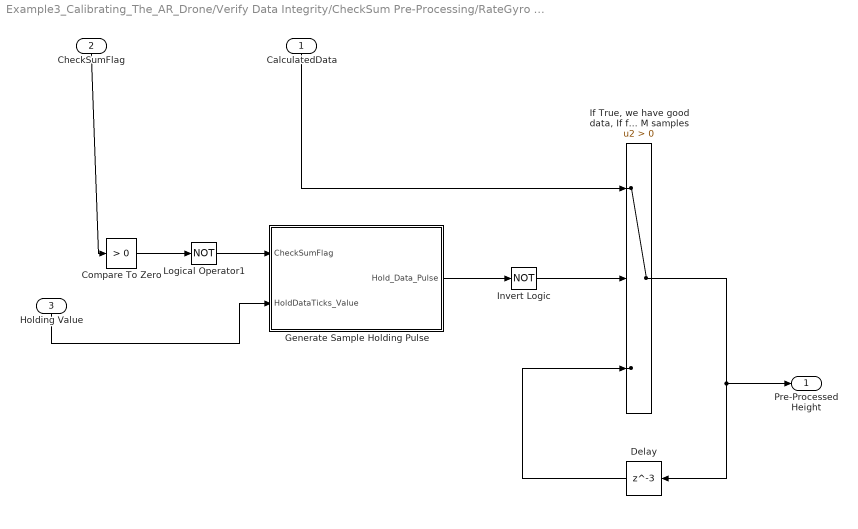
== system Example3_Calibrating_The_AR_Drone/Verify Data Integrity/CheckSum Pre-Processing/RateGyro Processing/CheckSum Correction ==
  CalculatedData : Inport
  CheckSumFlag : Inport  Port=2
  Holding Value : Inport  Port=3
  Compare To Zero : simulink/Logic and Bit Operations/Compare To Zero  relop=>  OutDataTypeStr=boolean
  Delay : Delay  DelayLength=3  InitialCondition=0
  Generate Sample Holding Pulse : Subsystem
  "If True, we have good data, If false, we have bad data, With bad data, use previous good data from N samples ago and hold it on that value for M samples" : Switch  Criteria=u2 > Threshold
  Invert Logic : Logic  Operator=NOT  AllPortsSameDT=off  OutDataTypeStr=boolean
  Logical Operator1 : Logic  Operator=NOT  AllPortsSameDT=off  OutDataTypeStr=boolean
  Pre-Processed Height : Outport
  wires:
  Holding Value/1 -> Generate Sample Holding Pulse/2(HoldDataTicks_Value)
  Invert Logic/1 -> "If True, we have good data, If false, we have bad data, With bad data, use previous good data from N samples ago and hold it on that value for M samples"/2
  Logical Operator1/1 -> Generate Sample Holding Pulse/1(CheckSumFlag)
  Generate Sample Holding Pulse/1(Hold_Data_Pulse) -> Invert Logic/1
  Compare To Zero/1 -> Logical Operator1/1
  Delay/1 -> "If True, we have good data, If false, we have bad data, With bad data, use previous good data from N samples ago and hold it on that value for M samples"/3
  "If True, we have good data, If false, we have bad data, With bad data, use previous good data from N samples ago and hold it on that value for M samples"/1 -> Delay/1, Pre-Processed Height/1
  CalculatedData/1 -> "If True, we have good data, If false, we have bad data, With bad data, use previous good data from N samples ago and hold it on that value for M samples"/1
  CheckSumFlag/1 -> Compare To Zero/1

== system Example3_Calibrating_The_AR_Drone/Verify Data Integrity/CheckSum Pre-Processing/RateGyro Processing/Process Data ==
  note: const float Sensitivity[ 3 ] = { 0.0609 , 0.0609 , 0.0609 } ;
      | const float Neutral[ 3 ] = { 0.0 , 0.0 , 0.0 } ;
      | const int16_t Offset[ 3 ] = { - 73 , 14 , - 13 } ;
      | const int16_t Noises[ 3 ] = { 35 , 35 , 15 } ;
      |
      | int16_t vRaws[ 3 ] = {
      | Navdata :: IMU :: Gyroscope :: getRawX (),
      | Navdata :: IMU :: Gyroscope :: getRawY (),
      | Navdata :: IMU :: Gyroscope :: getRawZ ()
      | } ;
      |
      | gyroscope[i] = vRaws[i] * Gyroscope :: Sensitivity[i] * M_PI / 180.0 ;
  Raw Data : Inport
  Constant : Constant  Value=[0.0, 0.0, 0.0]
  Gain : Gain  Gain=[0.0609, 0.0609, 0.0609]
  Sum : Sum  Inputs=|++
  Processed Data : Outport
  wires:
  Raw Data/1 -> Sum/1
  Constant/1 -> Sum/2
  Gain/1 -> Processed Data/1
  Sum/1 -> Gain/1

== system Example3_Calibrating_The_AR_Drone/Verify Data Integrity/CheckSum Pre-Processing/TempFilter/CheckSum Correction ==
  CalculatedData : Inport
  CheckSumFlag : Inport  Port=2
  Holding Value : Inport  Port=3
  Compare To Zero : simulink/Logic and Bit Operations/Compare To Zero  relop=>  OutDataTypeStr=boolean
  Delay : Delay  DelayLength=3  InitialCondition=0
  Generate Sample Holding Pulse : Subsystem
  "If True, we have good data, If false, we have bad data, With bad data, use previous good data from N samples ago and hold it on that value for M samples" : Switch  Criteria=u2 > Threshold
  Invert Logic : Logic  Operator=NOT  AllPortsSameDT=off  OutDataTypeStr=boolean
  Logical Operator1 : Logic  Operator=NOT  AllPortsSameDT=off  OutDataTypeStr=boolean
  Pre-Processed Data : Outport
  wires:
  Holding Value/1 -> Generate Sample Holding Pulse/2(HoldDataTicks_Value)
  Invert Logic/1 -> "If True, we have good data, If false, we have bad data, With bad data, use previous good data from N samples ago and hold it on that value for M samples"/2
  Logical Operator1/1 -> Generate Sample Holding Pulse/1(CheckSumFlag)
  Generate Sample Holding Pulse/1(Hold_Data_Pulse) -> Invert Logic/1
  Compare To Zero/1 -> Logical Operator1/1
  Delay/1 -> "If True, we have good data, If false, we have bad data, With bad data, use previous good data from N samples ago and hold it on that value for M samples"/3
  "If True, we have good data, If false, we have bad data, With bad data, use previous good data from N samples ago and hold it on that value for M samples"/1 -> Delay/1, Pre-Processed Data/1
  CalculatedData/1 -> "If True, we have good data, If false, we have bad data, With bad data, use previous good data from N samples ago and hold it on that value for M samples"/1
  CheckSumFlag/1 -> Compare To Zero/1

== system Example3_Calibrating_The_AR_Drone/Verify Data Integrity/CheckSum Pre-Processing/TempFilter/Process Raw Mag Data ==
  note: magnetometer[ 0 ] = - ( float ) navdata.mx ;
      | magnetometer[ 1 ] = ( float ) navdata.my ;
      | magnetometer[ 2 ] = - ( float ) navdata.mz ;
      | const float Sensitivity[ 3 ] = { 0.0071492608 , 0.0070882491 , 0.0074057781 } ;
      | const float Neutral[ 3 ] = { 118.0 , - 65.0 , 110.0 } ;
  Magnetometer : Inport
  Bias : Constant  Value=[ 118.0, -65.0, 110.0 ]
  Sum : Sum  Inputs=|+-
  postGain : Gain  Gain=[0.0071492608, 0.0070882491, 0.0074057781]
  preGain : Gain  Gain=[-1 1 -1]
  ProcessedData : Outport
  wires:
  Bias/1 -> Sum/2
  preGain/1 -> Sum/1
  Sum/1 -> postGain/1
  Magnetometer/1 -> preGain/1
  postGain/1 -> ProcessedData/1

== system Example3_Calibrating_The_AR_Drone/Verify Data Integrity/CheckSum Pre-Processing/Ultrasound Processing/CheckSum Correction ==
  CalculatedData : Inport
  CheckSumFlag : Inport  Port=2
  Holding Value : Inport  Port=3
  Compare To Zero : simulink/Logic and Bit Operations/Compare To Zero  relop=>  OutDataTypeStr=boolean
  Delay : Delay  DelayLength=3  InitialCondition=0
  Generate Sample Holding Pulse : Subsystem
  "If True, we have good data, If false, we have bad data, With bad data, use previous good data from N samples ago and hold it on that value for M samples" : Switch  Criteria=u2 > Threshold
  Invert Logic : Logic  Operator=NOT  AllPortsSameDT=off  OutDataTypeStr=boolean
  Logical Operator1 : Logic  Operator=NOT  AllPortsSameDT=off  OutDataTypeStr=boolean
  Pre-Processed Height : Outport
  wires:
  Holding Value/1 -> Generate Sample Holding Pulse/2(HoldDataTicks_Value)
  Invert Logic/1 -> "If True, we have good data, If false, we have bad data, With bad data, use previous good data from N samples ago and hold it on that value for M samples"/2
  Logical Operator1/1 -> Generate Sample Holding Pulse/1(CheckSumFlag)
  Generate Sample Holding Pulse/1(Hold_Data_Pulse) -> Invert Logic/1
  Compare To Zero/1 -> Logical Operator1/1
  Delay/1 -> "If True, we have good data, If false, we have bad data, With bad data, use previous good data from N samples ago and hold it on that value for M samples"/3
  "If True, we have good data, If false, we have bad data, With bad data, use previous good data from N samples ago and hold it on that value for M samples"/1 -> Delay/1, Pre-Processed Height/1
  CalculatedData/1 -> "If True, we have good data, If false, we have bad data, With bad data, use previous good data from N samples ago and hold it on that value for M samples"/1
  CheckSumFlag/1 -> Compare To Zero/1

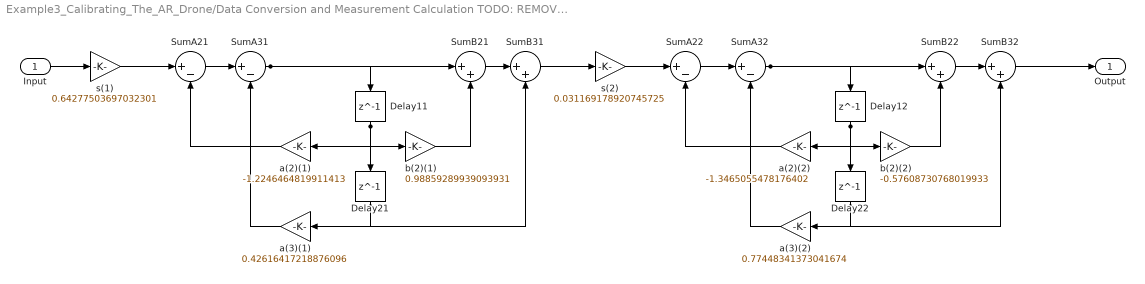
== system Example3_Calibrating_The_AR_Drone/Data Conversion and Measurement Calculation TODO: REMOVE // SIMPLIFY THIS?/Calibration_Scale_and_Offset/Process Raw Mag Data/Process Raw Mag Data (Work_255725)/Low Pass Filter1 ==
  Input : Inport
  Delay{11..12,21..22} (4 alike) : Delay  DelayLength=1  InitialCondition=0
  SumA{21..22,31..32} (4 alike) : Sum  Inputs=|+-  RndMeth=Nearest  SaturateOnIntegerOverflow=on  OutDataTypeStr=Inherit: Same as first input
  SumB{21..22,31..32} (4 alike) : Sum  Inputs=|++  RndMeth=Nearest  SaturateOnIntegerOverflow=on  OutDataTypeStr=Inherit: Same as first input
  a(2)(1) : Gain  Gain=-1.2246464819911413  ParamDataTypeStr=double  RndMeth=Nearest  SaturateOnIntegerOverflow=on  OutDataTypeStr=Inherit: Same as input
  a(2)(2) : Gain  Gain=-1.3465055478176402  ParamDataTypeStr=double  RndMeth=Nearest  SaturateOnIntegerOverflow=on  OutDataTypeStr=Inherit: Same as input
  a(3)(1) : Gain  Gain=0.42616417218876096  ParamDataTypeStr=double  RndMeth=Nearest  SaturateOnIntegerOverflow=on  OutDataTypeStr=Inherit: Same as input
  a(3)(2) : Gain  Gain=0.77448341373041674  ParamDataTypeStr=double  RndMeth=Nearest  SaturateOnIntegerOverflow=on  OutDataTypeStr=Inherit: Same as input
  b(2)(1) : Gain  Gain=0.98859289939093931  ParamDataTypeStr=double  RndMeth=Nearest  SaturateOnIntegerOverflow=on  OutDataTypeStr=Inherit: Same as input
  b(2)(2) : Gain  Gain=-0.57608730768019933  ParamDataTypeStr=double  RndMeth=Nearest  SaturateOnIntegerOverflow=on  OutDataTypeStr=Inherit: Same as input
  s(1) : Gain  Gain=0.64277503697032301  ParamDataTypeStr=double  RndMeth=Nearest  SaturateOnIntegerOverflow=on  OutDataTypeStr=Inherit: Same as input
  s(2) : Gain  Gain=0.031169178920745725  ParamDataTypeStr=double  RndMeth=Nearest  SaturateOnIntegerOverflow=on  OutDataTypeStr=Inherit: Same as input
  Output : Outport
  wires:
  Delay22/1 -> SumB32/2, a(3)(2)/1
  a(3)(2)/1 -> SumA32/2
  b(2)(2)/1 -> SumB22/2
  Delay12/1 -> Delay22/1, b(2)(2)/1, a(2)(2)/1
  a(2)(2)/1 -> SumA22/2
  SumB32/1 -> Output/1
  SumB22/1 -> SumB32/1
  SumA32/1 -> Delay12/1, SumB22/1
  SumA22/1 -> SumA32/1
  s(2)/1 -> SumA22/1
  Delay21/1 -> SumB31/2, a(3)(1)/1
  a(3)(1)/1 -> SumA31/2
  b(2)(1)/1 -> SumB21/2
  Delay11/1 -> Delay21/1, b(2)(1)/1, a(2)(1)/1
  a(2)(1)/1 -> SumA21/2
  SumB31/1 -> s(2)/1
  SumB21/1 -> SumB31/1
  SumA31/1 -> Delay11/1, SumB21/1
  SumA21/1 -> SumA31/1
  s(1)/1 -> SumA21/1
  Input/1 -> s(1)/1

== system Example3_Calibrating_The_AR_Drone/Verify Data Integrity/CheckSum Pre-Processing/Accelerometer Processing/CheckSum Correction/Generate Sample Holding Pulse ==
  CheckSumFlag : Inport
  HoldDataTicks_Value : Inport  Port=2
  Chart : Stateflow chart  TreatAsAtomicUnit=on
  Constant2 : Constant
  Logical Operator1 : Logic  AllPortsSameDT=off  OutDataTypeStr=boolean
  Transition Logic Detection : Subsystem
  Hold_Data_Pulse : Outport
  wires:
  HoldDataTicks_Value/1 -> Chart/2(HoldDataTicks)
  CheckSumFlag/1 -> Transition Logic Detection/1(Input)
  Transition Logic Detection/1(Transition Detect) -> Chart/1(if_transition)
  Chart/1(output) -> Logical Operator1/2
  Logical Operator1/1 -> Hold_Data_Pulse/1
  Constant2/1 -> Logical Operator1/1

== system Example3_Calibrating_The_AR_Drone/Verify Data Integrity/CheckSum Pre-Processing/Magnetometer/CheckSum Correction/Generate Sample Holding Pulse ==
  CheckSumFlag : Inport
  HoldDataTicks_Value : Inport  Port=2
  Chart : Stateflow chart  TreatAsAtomicUnit=on
  Constant2 : Constant
  Logical Operator1 : Logic  AllPortsSameDT=off  OutDataTypeStr=boolean
  Transition Logic Detection : Subsystem
  Hold_Data_Pulse : Outport
  wires:
  HoldDataTicks_Value/1 -> Chart/2(HoldDataTicks)
  CheckSumFlag/1 -> Transition Logic Detection/1(Input)
  Transition Logic Detection/1(Transition Detect) -> Chart/1(if_transition)
  Chart/1(output) -> Logical Operator1/2
  Logical Operator1/1 -> Hold_Data_Pulse/1
  Constant2/1 -> Logical Operator1/1

== system Example3_Calibrating_The_AR_Drone/Verify Data Integrity/CheckSum Pre-Processing/RateGyro Processing/CheckSum Correction/Generate Sample Holding Pulse ==
  CheckSumFlag : Inport
  HoldDataTicks_Value : Inport  Port=2
  Chart : Stateflow chart  TreatAsAtomicUnit=on
  Constant2 : Constant
  Logical Operator1 : Logic  AllPortsSameDT=off  OutDataTypeStr=boolean
  Transition Logic Detection : Subsystem
  Hold_Data_Pulse : Outport
  wires:
  HoldDataTicks_Value/1 -> Chart/2(HoldDataTicks)
  CheckSumFlag/1 -> Transition Logic Detection/1(Input)
  Transition Logic Detection/1(Transition Detect) -> Chart/1(if_transition)
  Chart/1(output) -> Logical Operator1/2
  Logical Operator1/1 -> Hold_Data_Pulse/1
  Constant2/1 -> Logical Operator1/1

== system Example3_Calibrating_The_AR_Drone/Verify Data Integrity/CheckSum Pre-Processing/TempFilter/CheckSum Correction/Generate Sample Holding Pulse ==
  CheckSumFlag : Inport
  HoldDataTicks_Value : Inport  Port=2
  Chart : Stateflow chart  TreatAsAtomicUnit=on
  Constant2 : Constant
  Logical Operator1 : Logic  AllPortsSameDT=off  OutDataTypeStr=boolean
  Transition Logic Detection : Subsystem
  Hold_Data_Pulse : Outport
  wires:
  HoldDataTicks_Value/1 -> Chart/2(HoldDataTicks)
  CheckSumFlag/1 -> Transition Logic Detection/1(Input)
  Transition Logic Detection/1(Transition Detect) -> Chart/1(if_transition)
  Chart/1(output) -> Logical Operator1/2
  Logical Operator1/1 -> Hold_Data_Pulse/1
  Constant2/1 -> Logical Operator1/1

== system Example3_Calibrating_The_AR_Drone/Verify Data Integrity/CheckSum Pre-Processing/Ultrasound Processing/CheckSum Correction/Generate Sample Holding Pulse ==
  CheckSumFlag : Inport
  HoldDataTicks_Value : Inport  Port=2
  Chart : Stateflow chart  TreatAsAtomicUnit=on
  Constant2 : Constant
  Logical Operator1 : Logic  AllPortsSameDT=off  OutDataTypeStr=boolean
  Transition Logic Detection : Subsystem
  Hold_Data_Pulse : Outport
  wires:
  HoldDataTicks_Value/1 -> Chart/2(HoldDataTicks)
  CheckSumFlag/1 -> Transition Logic Detection/1(Input)
  Transition Logic Detection/1(Transition Detect) -> Chart/1(if_transition)
  Chart/1(output) -> Logical Operator1/2
  Logical Operator1/1 -> Hold_Data_Pulse/1
  Constant2/1 -> Logical Operator1/1

== system Example3_Calibrating_The_AR_Drone/Verify Data Integrity/CheckSum Pre-Processing/Accelerometer Processing/CheckSum Correction/Generate Sample Holding Pulse/Transition Logic Detection ==
  Input : Inport
  Constant : Constant  Value=0
  Constant1 : Constant
  Logical Operator : Logic  AllPortsSameDT=off  OutDataTypeStr=boolean
  Relational Operator : RelationalOperator  Operator===  OutDataTypeStr=boolean
  Relational Operator1 : RelationalOperator  Operator===  OutDataTypeStr=boolean
  Unit Delay : UnitDelay  SampleTime=-1
  Transition Detect : Outport
  wires:
  Logical Operator/1 -> Transition Detect/1  "Transition_Detect"
  Constant1/1 -> Relational Operator1/1
  Constant/1 -> Relational Operator/2
  Relational Operator/1 -> Logical Operator/2
  Input/1 -> Unit Delay/1, Relational Operator1/2
  Unit Delay/1 -> Relational Operator/1
  Relational Operator1/1 -> Logical Operator/1

== system Example3_Calibrating_The_AR_Drone/Verify Data Integrity/CheckSum Pre-Processing/Magnetometer/CheckSum Correction/Generate Sample Holding Pulse/Transition Logic Detection ==
  Input : Inport
  Constant : Constant  Value=0
  Constant1 : Constant
  Logical Operator : Logic  AllPortsSameDT=off  OutDataTypeStr=boolean
  Relational Operator : RelationalOperator  Operator===  OutDataTypeStr=boolean
  Relational Operator1 : RelationalOperator  Operator===  OutDataTypeStr=boolean
  Unit Delay : UnitDelay  SampleTime=-1
  Transition Detect : Outport
  wires:
  Logical Operator/1 -> Transition Detect/1  "Transition_Detect"
  Constant1/1 -> Relational Operator1/1
  Constant/1 -> Relational Operator/2
  Relational Operator/1 -> Logical Operator/2
  Input/1 -> Unit Delay/1, Relational Operator1/2
  Unit Delay/1 -> Relational Operator/1
  Relational Operator1/1 -> Logical Operator/1

== system Example3_Calibrating_The_AR_Drone/Verify Data Integrity/CheckSum Pre-Processing/RateGyro Processing/CheckSum Correction/Generate Sample Holding Pulse/Transition Logic Detection ==
  Input : Inport
  Constant : Constant  Value=0
  Constant1 : Constant
  Logical Operator : Logic  AllPortsSameDT=off  OutDataTypeStr=boolean
  Relational Operator : RelationalOperator  Operator===  OutDataTypeStr=boolean
  Relational Operator1 : RelationalOperator  Operator===  OutDataTypeStr=boolean
  Unit Delay : UnitDelay  SampleTime=-1
  Transition Detect : Outport
  wires:
  Logical Operator/1 -> Transition Detect/1  "Transition_Detect"
  Constant1/1 -> Relational Operator1/1
  Constant/1 -> Relational Operator/2
  Relational Operator/1 -> Logical Operator/2
  Input/1 -> Unit Delay/1, Relational Operator1/2
  Unit Delay/1 -> Relational Operator/1
  Relational Operator1/1 -> Logical Operator/1

== system Example3_Calibrating_The_AR_Drone/Verify Data Integrity/CheckSum Pre-Processing/TempFilter/CheckSum Correction/Generate Sample Holding Pulse/Transition Logic Detection ==
  Input : Inport
  Constant : Constant  Value=0
  Constant1 : Constant
  Logical Operator : Logic  AllPortsSameDT=off  OutDataTypeStr=boolean
  Relational Operator : RelationalOperator  Operator===  OutDataTypeStr=boolean
  Relational Operator1 : RelationalOperator  Operator===  OutDataTypeStr=boolean
  Unit Delay : UnitDelay  SampleTime=-1
  Transition Detect : Outport
  wires:
  Logical Operator/1 -> Transition Detect/1  "Transition_Detect"
  Constant1/1 -> Relational Operator1/1
  Constant/1 -> Relational Operator/2
  Relational Operator/1 -> Logical Operator/2
  Input/1 -> Unit Delay/1, Relational Operator1/2
  Unit Delay/1 -> Relational Operator/1
  Relational Operator1/1 -> Logical Operator/1

== system Example3_Calibrating_The_AR_Drone/Verify Data Integrity/CheckSum Pre-Processing/Ultrasound Processing/CheckSum Correction/Generate Sample Holding Pulse/Transition Logic Detection ==
  Input : Inport
  Constant : Constant  Value=0
  Constant1 : Constant
  Logical Operator : Logic  AllPortsSameDT=off  OutDataTypeStr=boolean
  Relational Operator : RelationalOperator  Operator===  OutDataTypeStr=boolean
  Relational Operator1 : RelationalOperator  Operator===  OutDataTypeStr=boolean
  Unit Delay : UnitDelay  SampleTime=-1
  Transition Detect : Outport
  wires:
  Logical Operator/1 -> Transition Detect/1  "Transition_Detect"
  Constant1/1 -> Relational Operator1/1
  Constant/1 -> Relational Operator/2
  Relational Operator/1 -> Logical Operator/2
  Input/1 -> Unit Delay/1, Relational Operator1/2
  Unit Delay/1 -> Relational Operator/1
  Relational Operator1/1 -> Logical Operator/1

== matlab function Example3_Calibrating_The_AR_Drone/Euler Angles/Compute Euler Angles/Compute euler angles from accelerometer ==
  data: Ax_Ay_Az input; Roll output; Pitch output
function [Roll,Pitch] = CalculateAngle(Ax_Ay_Az)

% using the method as described in
% http://www.digikey.com/en/articles/techzone/2011/may/using-an-accelerometer-for-inclination-sensing
%#codegen
Ax = -Ax_Ay_Az(1);
Ay = -Ax_Ay_Az(2);
Az = Ax_Ay_Az(3);

Roll = 180 / pi * atan( Ay / sqrt( Ax^2 + Az^2));
Pitch = -180 / pi * atan( Ax / sqrt( Ay^2 + Az^2));

== stateflow chart Example3_Calibrating_The_AR_Drone/Verify Data Integrity/CheckSum Pre-Processing/Accelerometer Processing/CheckSum Correction/Generate Sample Holding Pulse/Chart ==
  state Begin_State0
    entry: output =0;
  state Begin_State
    entry: output =1;
  state End_State
    entry: output=0;
  (default) -> Begin_State0
  Begin_State0 -> Begin_State : [if_transition==1]
  Begin_State -> End_State [order 1] : after(HoldDataTicks,tick)
  End_State -> Begin_State : [if_transition==1]
  Begin_State -> Begin_State [order 2] : [if_transition==1]
  data: output output; if_transition input; HoldDataTicks input

== stateflow chart Example3_Calibrating_The_AR_Drone/Verify Data Integrity/CheckSum Pre-Processing/Magnetometer/CheckSum Correction/Generate Sample Holding Pulse/Chart ==
  state Begin_State0
    entry: output =0;
  state Begin_State
    entry: output =1;
  state End_State
    entry: output=0;
  (default) -> Begin_State0
  Begin_State0 -> Begin_State : [if_transition==1]
  Begin_State -> End_State [order 1] : after(HoldDataTicks,tick)
  End_State -> Begin_State : [if_transition==1]
  Begin_State -> Begin_State [order 2] : [if_transition==1]
  data: output output; if_transition input; HoldDataTicks input

== stateflow chart Example3_Calibrating_The_AR_Drone/Verify Data Integrity/CheckSum Pre-Processing/RateGyro Processing/CheckSum Correction/Generate Sample Holding Pulse/Chart ==
  state Begin_State0
    entry: output =0;
  state Begin_State
    entry: output =1;
  state End_State
    entry: output=0;
  (default) -> Begin_State0
  Begin_State0 -> Begin_State : [if_transition==1]
  Begin_State -> End_State [order 1] : after(HoldDataTicks,tick)
  End_State -> Begin_State : [if_transition==1]
  Begin_State -> Begin_State [order 2] : [if_transition==1]
  data: output output; if_transition input; HoldDataTicks input

== stateflow chart Example3_Calibrating_The_AR_Drone/Verify Data Integrity/CheckSum Pre-Processing/TempFilter/CheckSum Correction/Generate Sample Holding Pulse/Chart ==
  state Begin_State0
    entry: output =0;
  state Begin_State
    entry: output =1;
  state End_State
    entry: output=0;
  (default) -> Begin_State0
  Begin_State0 -> Begin_State : [if_transition==1]
  Begin_State -> End_State [order 1] : after(HoldDataTicks,tick)
  End_State -> Begin_State : [if_transition==1]
  Begin_State -> Begin_State [order 2] : [if_transition==1]
  data: output output; if_transition input; HoldDataTicks input

== stateflow chart Example3_Calibrating_The_AR_Drone/Verify Data Integrity/CheckSum Pre-Processing/Ultrasound Processing/CheckSum Correction/Generate Sample Holding Pulse/Chart ==
  state Begin_State0
    entry: output =0;
  state Begin_State
    entry: output =1;
  state End_State
    entry: output=0;
  (default) -> Begin_State0
  Begin_State0 -> Begin_State : [if_transition==1]
  Begin_State -> End_State [order 1] : after(HoldDataTicks,tick)
  End_State -> Begin_State : [if_transition==1]
  Begin_State -> Begin_State [order 2] : [if_transition==1]
  data: output output; if_transition input; HoldDataTicks input

== matlab function Example3_Calibrating_The_AR_Drone/Verify Data Integrity/CheckSum Pre-Processing/Ultrasound Processing/Height Calculation ==
  data: u input double; y output double; prev_good_height output double; z_1 input double
function [y,prev_good_height] = fcn(u,z_1)
%#codegen



if u<10000
    
    height = ((u - 880) /26.553);
    prev_good_height = height;
else
    
%     height = u;
%     prev_good_height = height;
    height =  z_1;
    prev_good_height = z_1; 
end

y = height;
